simulink model "pickAndPlaceSequence"  (R2019b)
settings: Solver=ode23t  StartTime=0.0  StopTime=40  FixedStep=0.01  MaxStep=0.05  RelTol=1e-3  EnableMultiTasking=on
PreLoadFcn:
  | mdl_puma560
values from neighbouring files (symbols this model uses):
  R = SerialLink(L, 'name', '210F', 'comment', 'six DOF', 'manufacturer', 'FANUC')    [Model_210F.m]
undefined symbols (not defined in the file or in its folder): slcoulomb
libraries: roblocks x14, simulink x7
settings Model: ExtModeTrigMode=oneshot  ExtModeArmWhenConnect=off  Creator=pic  LastModifiedBy=Karl
settings SolverCC: ZeroCrossControl=DisableAll
settings DataIOCC: SaveFormat=Array  SignalLoggingSaveFormat=ModelDataLogs  TimeSaveName=t  OutputSaveName=y  ReturnWorkspaceOutputsName=Rsim
settings OptimizationCC: BlockReduction=off  BooleanDataType=off  ExpressionDepthLimit=2147483647  InitFltsAndDblsToZero=on  LifeSpan=inf
settings DebuggingCC: SaveWithParameterizedLinksMsg=none  UnderspecifiedInitializationDetection=Classic  MergeDetectMultiDrivingBlocksExec=none  SignalResolutionControl=TryResolveAllWithWarning  MultiTaskDSMMsg=warning  MultiTaskCondExecSysMsg=none  FcnCallInpInsideContextMsg=warning  AllowSymbolicDim=off  StateNameClashWarn=warning  SFUnexpectedBacktrackingDiag=warning  SFNoUnconditionalDefaultTransitionDiag=warning  SFExecutionAtInitializationDiag=none  ArithmeticOperatorsInVariantConditions=warning
settings HardwareCC: ProdBitPerPointer=32  ProdBitPerSizeT=32  ProdBitPerPtrDiffT=32  ProdLargestAtomicFloat=None  ProdIntDivRoundTo=Undefined  ProdEndianess=Unspecified  ProdWordSize=32  ProdHWDeviceType=32-bit Generic  TargetUnknown=on
settings ModelReferenceCC: PropagateSignalLabelsOutOfModel=off
settings SFSimCC: SimUseLocalCustomCode=off  CustomCodeUndefinedFunction=UseInterfaceOnly
settings RTWCC: RTWUseLocalCustomCode=off
settings CodeAppCC: StateflowObjectComments=on
settings GRTTargetCC: TargetLangStandard=C89/C90 (ANSI)  ModelReferenceCompliant=off  CompOptLevelCompliant=off  GeneratePreprocessorConditionals=Disable all  CombineOutputUpdateFcns=off  MatFileLogging=off  GRTInterface=on
settings ConfigComp: CovMetricSettings=dw  CovHtmlReporting=on  CovSaveCumulativeToWorkspaceVar=on  CovSaveSingleToWorkspaceVar=on  CovExternalEMLEnable=off

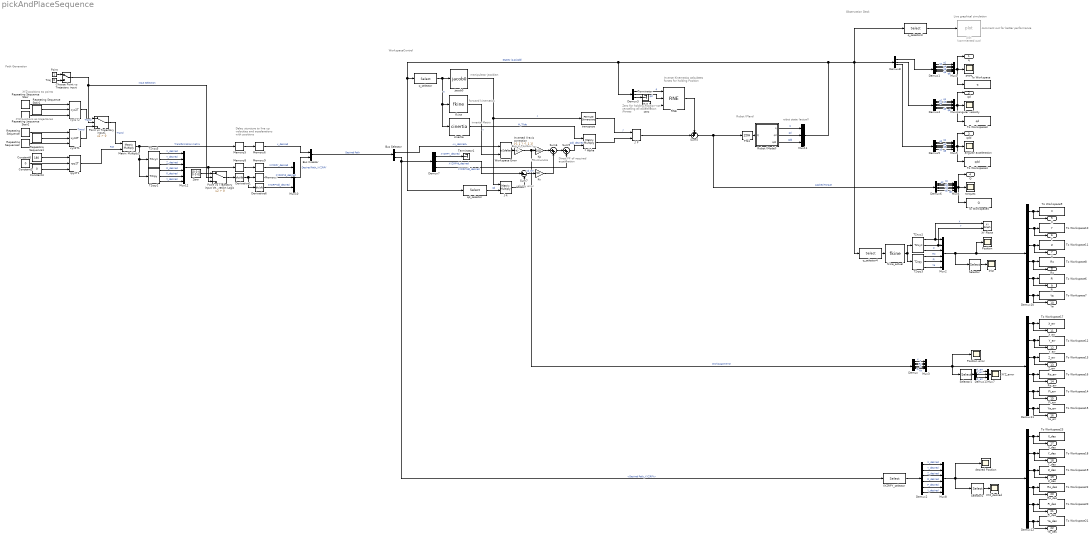
== system pickAndPlaceSequence ==
  note: Live graphical simulation
  note: comment out for better performance
  note: manipulator jacobian
  note: innertia Matrix
  note: forward kinematics
  note: XYZ positions as trajectories
  note: XYZ-positions as points
  note: Delay sturcture to line up velocities and accelerations with positions
  note: position error
  note: velocity error
  note: Direct FF
      | of required
      |  acceleration
  note: PD-strucutre
  note: Inverse Kinematics
      | calculates forces
      | for holding Position
  note: Bug in Toolbox!
  note: WorkspaceControl
  note: Zero for
      | holding Position
      | not cancelling
      | all acceleration
      | /forces
  note: Robot (Plant)
  note: robot state
      | (actual)
  note: Path Generation
  note: Observation Deck
  "* Alpha " : Product  Multiplication=Matrix(*)
  Bus Creator : BusCreator  Inputs=2
  Bus Selector : BusSelector  OutputSignals=x_desired,Desired Path_XYZRPY
  Choose Point vs Trajectory input : ManualSwitch
  Constant1 : Constant  Value=0
  Constant4 : Constant  Value=0
  Constant6 : Constant  Value=180
  Demux{,1..2,4..6,10..12} (9 alike) : Demux  Outputs=6
  Demux{3,7..8,13} (4 alike) : Demux  Outputs=3
  Derivative1 : Derivative
  Derivative6 : Derivative
  "Inverted X-axis correction " : Gain  Gain=[-1 1 1 -1 1 1]
  J q : Product  Multiplication=Matrix(*)
  J' F : Product  Multiplication=Matrix(*)
  Kp : Gain  Gain=100
  Kv : Gain  Gain=50
  Matrix Multiply1 : Product  Multiplication=Matrix(*)
  Memory5 : Memory  InitialCondition=eye(4)  InheritSampleTime=on
  Memory6 : Memory  InitialCondition=eye(4)  InheritSampleTime=on
  Memory7 : Memory  InitialCondition=[0 0 0 0 0 0]  InheritSampleTime=on
  Memory8 : Memory  InitialCondition=[0 0 0 0 0 0]  InheritSampleTime=on
  Memory9 : Memory  InitialCondition=[0 0 0 0 0 0]  InheritSampleTime=on
  Mux{1..6,8,12} (8 alike) : Mux  Inputs=6
  Mux10 : Mux  Inputs=3
  Mux11 : Mux  Inputs=3
  Mux7 : Mux  Inputs=3
  Point : Constant
  Point vs Trajectory input Velocity/Acceleration Logic : Switch  Criteria=u2 > Threshold
  Point vs Trajectory input1 : Switch  Criteria=u2 > Threshold
  Position : Scope
  Position error : Scope
  RNE : roblocks/Arm/RNE  robot=R.nofriction  grav=[0 0 9.81]
  Repeating Sequence : simulink/Sources/Repeating Sequence  rep_seq_t=[0 2 4 6 8 10 12 14 16 18 20 22 24 26 28 30 32]  rep_seq_y=[0.9 0.9 0.9 0.9 1.850 2.250 2.250 2 1.650 2.250 2.250 1.250 0.815 0.815 0.815 0.885 0.9 ]
  Repeating Sequence Stair : simulink/Sources/Repeating Sequence Stair  OutValues=[0.9 0.9 0.9 0.9 1.850 2.250 2.250 2 1.650 2.250 2.250 1.250 0.815 0.815 0.815 0.885 0.9 ]  tsamp=2  OutMin=[]  OutMax=[]  OutDataTypeStr=double  OutputDataTypeScalingMode=double  OutDataType=fixdt(0,8)  ConRadixGroup=Best Precision: Vector-wise  OutScaling=2^-12
  Repeating Sequence Stair1 : simulink/Sources/Repeating Sequence Stair  OutValues=[1.6 1.6 1.6 1 0 0 0 0 0 0 0 0 -1.695 -1.695 -1.695 0.5 1.6]  tsamp=2  OutMin=[]  OutMax=[]  OutDataTypeStr=double  OutputDataTypeScalingMode=double  OutDataType=fixdt(0,8)  ConRadixGroup=Best Precision: Vector-wise  OutScaling=2^-12
  Repeating Sequence Stair2 : simulink/Sources/Repeating Sequence Stair  OutValues=[0.026 -0.05 0.026 0.026 0.14 0.123 0.084 0.13 0.13 0.13 0.155 0.180 -0.17 -0.26 -0.17 0.026 0.026]  tsamp=2  OutMin=[]  OutMax=[]  OutDataTypeStr=double  OutputDataTypeScalingMode=double  OutDataType=fixdt(0,8)  ConRadixGroup=Best Precision: Vector-wise  OutScaling=2^-12
  Repeating Sequence1 : simulink/Sources/Repeating Sequence  rep_seq_t=[0 2 4 6 8 10 12 14 16 18 20 22 24 26 28 30 32]  rep_seq_y=[1.6 1.6 1.6 1 0 0 0 0 0 0 0 0 -1.695 -1.695 -1.695 0.5 1.6]
  Repeating Sequence2 : simulink/Sources/Repeating Sequence  rep_seq_t=[0 2 4 6 8 10 12 14 16 18 20 22 24 26 28 30 32]  rep_seq_y=[0.026 -0.05 0.026 0.026 0.14 0.123 0.084 0.13 0.13 0.13 0.155 0.180 -0.17 -0.26 -0.17 0.026 0.026]
  Robot (Model) : Subsystem  AncestorBlock=roblocks/Arm/Robot  mask{robot=R.nofriction, q0=[0 -pi/4 0 0 -pi/4 0]}
      mask prompts: robot "Robot object"; q0 "Initial state"
      mask help: Rigid-body dynamic model of robot.
      mask init:
      | if isa(robot, 'SerialLink')
      |     rname = robot.name;
      |     %fprintf('**robot name is %s\n', rname);
      | else
      |     rname = '';
      |     n = 0
      | end
      mask Help:
      | Simulates the forward (direct) rigid-body dynamics of the robot described
      | by the given robot object.  For given applied joint torque/force it computes
      | the instaneous joint coordinates, velocities and acclerations.
      | 
      | 
      | <b>Parameters::</b>
      | 
      | robot (SerialLink) a dynamic model of an N-link serial link manipulator
      | q0 (1xN)  Initial joint coordinates
      | 
      | <b>Inputs::</b>
      | 
      | Q (1xN) the generalized joint force (torque or force) required to achieve
      | the motion state (q, qd, qdd).
      | 
      | <b>Outputs::</b>
      | 
      | q (1xN) joint coordinates
      | qd (1xN) joint coordinate velocity
      | qdd (1xN) joint coordinate acceleration
      | 
      | 
      | <b>Notes::</b>
      | 
      | - Required to simulate robot rigid body motion.
      | - Implemented using the recursive Newton-Euler scheme (RNE).
      | - A wrapper for the Toolbox method accel() which in turn depends on the
      |   method rne().
      mask Display:
      | port_label('input', 1, 'Q')
      | port_label('output', 1, 'q')
      | port_label('output', 2, 'qd')
      | port_label('output', 3, 'qdd')
      | text(0.1, 0.9,  rname, 'horizontalAlignment', 'left')
  Selector : Selector  InputPortWidth=6  IndexOptions=Index vector (dialog)  Indices=[1 2 3]  OutputSizes=1
  Selector1 : Selector  InputPortWidth=6  IndexOptions=Index vector (dialog)  Indices=[1 2 3]  OutputSizes=1
  Selector2 : Selector  InputPortWidth=6  IndexOptions=Index vector (dialog)  Indices=[1 2 3]  OutputSizes=1
  Sum5 : Sum  Inputs=++|
  Sum6 : Sum  Inputs=|++
  Sum7 : Sum  Inputs=|+-
  Sum9 : Sum  Inputs=|++
  T2rpy2 : roblocks/Toolbox/T2rpy  sequence=ZYX  degrees=off
  T2rpy3 : roblocks/Toolbox/T2rpy  sequence=ZYX  degrees=off
  T2xyz1 : roblocks/Toolbox/T2xyz
  T2xyz3 : roblocks/Toolbox/T2xyz
  Terminator : Terminator
  Terminator1 : Terminator
  Tfb1 : ZeroOrderHold  SampleTime=0.005
  To Workspace : ToWorkspace  VariableName=q  SaveFormat=Timeseries  SampleTime=-1
  To Workspace10 : ToWorkspace  VariableName=Y  SaveFormat=Timeseries  SampleTime=-1
  To Workspace11 : ToWorkspace  VariableName=Z  SaveFormat=Timeseries  SampleTime=-1
  To Workspace12 : ToWorkspace  VariableName=Y_err  SaveFormat=Timeseries  SampleTime=-1
  To Workspace13 : ToWorkspace  VariableName=Z_err  SaveFormat=Timeseries  SampleTime=-1
  To Workspace14 : ToWorkspace  VariableName=Pi_err  SaveFormat=Timeseries  SampleTime=-1
  To Workspace15 : ToWorkspace  VariableName=Ya_err  SaveFormat=Timeseries  SampleTime=-1
  To Workspace16 : ToWorkspace  VariableName=Ro_err  SaveFormat=Timeseries  SampleTime=-1
  To Workspace17 : ToWorkspace  VariableName=X_err  SaveFormat=Timeseries  SampleTime=-1
  To Workspace18 : ToWorkspace  VariableName=Y_des  SaveFormat=Timeseries  SampleTime=-1
  To Workspace19 : ToWorkspace  VariableName=Z_des  SaveFormat=Timeseries  SampleTime=-1
  To Workspace20 : ToWorkspace  VariableName=Pi_des  SaveFormat=Timeseries  SampleTime=-1
  To Workspace21 : ToWorkspace  VariableName=Ya_des  SaveFormat=Timeseries  SampleTime=-1
  To Workspace22 : ToWorkspace  VariableName=Ro_des  SaveFormat=Timeseries  SampleTime=-1
  To Workspace23 : ToWorkspace  VariableName=X_des  SaveFormat=Timeseries  SampleTime=-1
  To Workspace3 : ToWorkspace  VariableName=qd  SaveFormat=Timeseries  SampleTime=-1
  To Workspace4 : ToWorkspace  VariableName=qdd  SaveFormat=Timeseries  SampleTime=-1
  To Workspace5 : ToWorkspace  VariableName=Q  SaveFormat=Timeseries  SampleTime=-1
  To Workspace6 : ToWorkspace  VariableName=Pi  SaveFormat=Timeseries  SampleTime=-1
  To Workspace7 : ToWorkspace  VariableName=Ya  SaveFormat=Timeseries  SampleTime=-1
  To Workspace8 : ToWorkspace  VariableName=Ro  SaveFormat=Timeseries  SampleTime=-1
  To Workspace9 : ToWorkspace  VariableName=X  SaveFormat=Timeseries  SampleTime=-1
  Traj : Constant  Value=0
  Workspace Error : roblocks/Toolbox/tr2delta
  XY Plane : simulink/Sinks/XY Graph  xmin=-3  xmax=3  ymin=-3  ymax=3  st=-1
  XYZ : Scope
  XYZRPY_selector : Selector  InputPortWidth=18  IndexOptions=Index vector (dialog)  Indices=[1 2 3 4 5 6]  OutputSizes=1
  XYZ_desired : Scope
  XYZ_error : Scope
  "Zero " : Constant  Value=[0 0 0 0 0 0]
  angular acceleration : Scope
  angular velocity : Scope
  "cinertia " : roblocks/Arm/cinertia  robot=R.nofriction
  desired Position : Scope
  "fkine " : roblocks/Arm/fkine  robot=R.nofriction
  fkine_actual : roblocks/Arm/fkine  robot=R.nofriction
  "jacob0 " : roblocks/Arm/jacob0   robot=R.nofriction
  plot : roblocks/Arm/plot  Commented=on  robot=R.nofriction  fps=10  holdplot=on
  pose : Scope
  q_selector : Selector  InputPortWidth=18  IndexOptions=Index vector (dialog)  Indices=[1 2 3 4 5 6]  OutputSizes=1
  q_selector3 : Selector  InputPortWidth=18  IndexOptions=Index vector (dialog)  Indices=[1 2 3 4 5 6]  OutputSizes=1
  q_selector4 : Selector  InputPortWidth=18  IndexOptions=Index vector (dialog)  Indices=[1 2 3 4 5 6]  OutputSizes=1
  qd_selector : Selector  InputPortWidth=18  IndexOptions=Index vector (dialog)  Indices=[7 8 9 10 11 12]  OutputSizes=1
  rpy2T1 : roblocks/Toolbox/rpy2T  sequence=ZYX  degrees=on
  torques : Scope
  transpose : PermuteDimensions
  xyz2T1 : roblocks/Toolbox/xyz2T
  xyz2T2 : roblocks/Toolbox/xyz2T
  zero : Constant  Value=[0 0 0 0 0 0]
  q : Outport  VectorParamsAs1DForOutWhenUnconnected=off
  qd : Outport  Port=2  VectorParamsAs1DForOutWhenUnconnected=off
  qdd : Outport  Port=3  VectorParamsAs1DForOutWhenUnconnected=off
  Q : Outport  Port=4  VectorParamsAs1DForOutWhenUnconnected=off
  X : Outport  Port=5  VectorParamsAs1DForOutWhenUnconnected=off
  Y : Outport  Port=6  VectorParamsAs1DForOutWhenUnconnected=off
  Z : Outport  Port=7
  Ro : Outport  Port=8  VectorParamsAs1DForOutWhenUnconnected=off
  Pi : Outport  Port=9  VectorParamsAs1DForOutWhenUnconnected=off
  Ya : Outport  Port=10
  X_err : Outport  Port=11  VectorParamsAs1DForOutWhenUnconnected=off
  Y_err : Outport  Port=12  VectorParamsAs1DForOutWhenUnconnected=off
  Z_err : Outport  Port=13
  Ro_err : Outport  Port=14  VectorParamsAs1DForOutWhenUnconnected=off
  Pi_err : Outport  Port=15  VectorParamsAs1DForOutWhenUnconnected=off
  Ya_err : Outport  Port=16
  X_des : Outport  Port=17  VectorParamsAs1DForOutWhenUnconnected=off
  Y_des : Outport  Port=18  VectorParamsAs1DForOutWhenUnconnected=off
  Z_des : Outport  Port=19
  Ro_des : Outport  Port=20  VectorParamsAs1DForOutWhenUnconnected=off
  Pi_des : Outport  Port=21  VectorParamsAs1DForOutWhenUnconnected=off
  Ya_des : Outport  Port=22
  wires:
  "jacob0 "/1 -> transpose/1, J q/1  "J"
  "fkine "/1 -> Workspace Error/2  "x"
  zero/1 -> RNE/3
  RNE/1 -> Sum5/1
  J' F/1 -> Sum5/2
  transpose/1 -> J' F/1  "J'"
  "* Alpha "/1 -> J' F/2
  Workspace Error/1 -> "Inverted X-axis correction "/1
  Kv/1 -> Sum6/2
  Sum7/1 -> Kv/1  "xd_err"
  Kp/1 -> Sum6/1
  J q/1 -> Sum7/2
  "cinertia "/1 -> "* Alpha "/1  "M_Tilde"
  Sum6/1 -> Sum9/1
  Demux7/2 -> Sum7/1  "XYZRPYd_desired"
  Sum9/1 -> "* Alpha "/2  "qdd_desired"
  Demux7/3 -> Sum9/2  "XYZRPYdd_desired"
  Memory6/1 -> Bus Creator/1  "x_desired"
  Robot (Model)/3(qdd) -> Mux11/3  "qdd"
  Robot (Model)/2(qd) -> Mux11/2  "qd"
  Robot (Model)/1(q) -> Mux11/1  "q"
  Tfb1/1 -> Robot (Model)/1(Q)
  Demux3/1 -> RNE/1  "q"
  Demux3/2 -> RNE/2  "qd"
  Demux3/3 -> Terminator/1
  qd_selector/1 -> J q/2  "qd"
  Memory8/1 -> Memory9/1
  Derivative1/1 -> Memory7/1, Derivative6/1
  Mux12/1 -> Point vs Trajectory input Velocity/Acceleration Logic/3, Memory8/1
  T2xyz3/2 -> Mux12/2  "Y_desired"
  T2xyz3/3 -> Mux12/3  "Z_desired"
  T2rpy2/2 -> Mux12/5  "P_desired"
  rpy2T1/1 -> Matrix Multiply1/2  "Rot"
  Matrix Multiply1/1 -> T2rpy2/1, T2xyz3/1, Memory5/1  "Transformation matrix"
  Derivative6/1 -> Mux10/3  "XYZRPYdd_desired"
  Memory7/1 -> Mux10/2  "XYZRPYd_desired"
  Point vs Trajectory input1/1 -> Matrix Multiply1/1  "Transl"
  T2rpy2/3 -> Mux12/6  "Y_desired"
  Memory5/1 -> Memory6/1
  Memory9/1 -> Mux10/1  "XYZRPY_desired"
  T2rpy2/1 -> Mux12/4  "R_desired"
  T2xyz3/1 -> Mux12/1  "X_desired"
  q_selector/1 -> "cinertia "/1, "fkine "/1, "jacob0 "/1  "q"
  Demux7/1 -> Terminator1/1  "XYZRPY_desired"
  Bus Selector/2 -> XYZRPY_selector/1, Demux7/1  "<Desired Path_XYZRPY>"
  Demux8/1 -> Demux1/1
  Mux7/1 -> XYZ_error/1
  Demux10/4 -> Ro/1, To Workspace8/1
  Demux10/2 -> Y/1, To Workspace10/1
  Mux11/1 -> Demux8/1, q_selector3/1, q_selector4/1, Demux3/1, qd_selector/1, q_selector/1  "States (q,qd,qdd)"
  q_selector4/1 -> fkine_actual/1
  fkine_actual/1 -> T2rpy3/1, T2xyz1/1
  Demux6/4 -> Mux6/4  "q4"
  Demux2/1 -> Mux8/1  "X_desired"
  Demux2/2 -> Mux8/2  "Y_desired"
  Demux4/3 -> Mux4/3  "q3"
  Demux2/6 -> Mux8/6  "Y_desired"
  Demux6/3 -> Mux6/3  "q3"
  Demux4/1 -> Mux4/1  "q1"
  Sum5/1 -> Tfb1/1, Demux6/1  "Applied Torque"
  Demux4/2 -> Mux4/2  "q2"
  Mux5/1 -> qdd/1, To Workspace4/1, angular acceleration/1
  Demux6/1 -> Mux6/1  "q1"
  Demux4/5 -> Mux4/5  "q5"
  Demux10/3 -> Z/1, To Workspace11/1
  Mux6/1 -> Q/1, To Workspace5/1, torques/1
  Demux6/5 -> Mux6/5  "q5"
  Demux6/6 -> Mux6/6  "q6"
  Demux5/1 -> Mux5/1  "q1"
  Demux10/6 -> Ya/1, To Workspace7/1
  Demux4/4 -> Mux4/4  "q4"
  Demux8/2 -> Demux4/1
  Demux5/6 -> Mux5/6  "q6"
  Demux5/4 -> Mux5/4  "q4"
  Demux1/5 -> Mux1/5  "q5"
  Demux4/6 -> Mux4/6  "q6"
  Demux1/1 -> Mux1/1  "q1"
  Mux1/1 -> q/1, To Workspace/1, pose/1
  Demux1/4 -> Mux1/4  "q4"
  Demux2/4 -> Mux8/4  "R_desired"
  Demux1/2 -> Mux1/2  "q2"
  Demux6/2 -> Mux6/2  "q2"
  Demux2/3 -> Mux8/3  "Z_desired"
  Demux5/3 -> Mux5/3  "q3"
  Demux5/2 -> Mux5/2  "q2"
  Demux2/5 -> Mux8/5  "P_desired"
  Demux1/3 -> Mux1/3  "q3"
  Demux1/6 -> Mux1/6  "q6"
  Selector1/1 -> Demux13/1
  Demux12/1 -> To Workspace23/1, X_des/1
  Demux12/5 -> Pi_des/1, To Workspace20/1
  Demux13/3 -> Mux7/3  "Z_err"
  Demux12/4 -> Ro_des/1, To Workspace22/1
  Demux11/5 -> Pi_err/1, To Workspace14/1
  Demux12/2 -> Y_des/1, To Workspace18/1
  Demux12/3 -> Z_des/1, To Workspace19/1
  Mux4/1 -> qd/1, To Workspace3/1, angular velocity/1
  Demux11/1 -> To Workspace17/1, X_err/1
  Demux11/4 -> Ro_err/1, To Workspace16/1
  Demux11/6 -> Ya_err/1, To Workspace15/1
  T2rpy3/1 -> Mux2/4  "Ro"
  T2rpy3/2 -> Mux2/5  "Pi"
  Demux11/3 -> Z_err/1, To Workspace13/1
  T2xyz1/3 -> Mux2/3  "Z"
  T2xyz1/2 -> XY Plane/2, Mux2/2  "Y"
  q_selector3/1 -> plot/1
  XYZRPY_selector/1 -> Demux2/1
  Selector2/1 -> XYZ_desired/1
  Demux12/6 -> Ya_des/1, To Workspace21/1
  Mux2/1 -> Position/1, Demux10/1, Selector/1
  Demux11/2 -> Y_err/1, To Workspace12/1
  Selector/1 -> XYZ/1
  Demux13/1 -> Mux7/1  "X_err"
  Demux8/3 -> Demux5/1
  Demux5/5 -> Mux5/5  "q5"
  T2rpy3/3 -> Mux2/6  "Ya"
  Demux13/2 -> Mux7/2  "Y_err"
  T2xyz1/1 -> XY Plane/1, Mux2/1  "X"
  Mux8/1 -> Demux12/1, Selector2/1, desired Position/1
  Demux10/5 -> Pi/1, To Workspace6/1
  Demux10/1 -> To Workspace9/1, X/1
  "Inverted X-axis correction "/1 -> Demux/1, Kp/1  "Workspace error"
  Demux/6 -> Mux3/6  "Ya"
  Demux/2 -> Mux3/2  "Y"
  Demux/4 -> Mux3/4  "Ro"
  Demux/5 -> Mux3/5  "Pi"
  Demux/1 -> Mux3/1  "X"
  Demux/3 -> Mux3/3  "Z"
  Mux3/1 -> Selector1/1, Position error/1, Demux11/1
  Bus Creator/1 -> Bus Selector/1  "Desired Path"
  Mux10/1 -> Bus Creator/2  "Desired Path_XYZRPY"
  Bus Selector/1 -> Workspace Error/1  "<x_desired>"
  Constant6/1 -> rpy2T1/1
  Constant1/1 -> rpy2T1/2
  Constant4/1 -> rpy2T1/3
  Repeating Sequence Stair2/1 -> xyz2T2/3
  Repeating Sequence Stair1/1 -> xyz2T2/2
  Repeating Sequence Stair/1 -> xyz2T2/1
  Repeating Sequence/1 -> xyz2T1/1
  Repeating Sequence2/1 -> xyz2T1/3
  Repeating Sequence1/1 -> xyz2T1/2
  xyz2T2/1 -> Point vs Trajectory input1/1  "Transl"
  xyz2T1/1 -> Point vs Trajectory input1/3  "Transl"
  Point vs Trajectory input Velocity/Acceleration Logic/1 -> Derivative1/1
  Point/1 -> Choose Point vs Trajectory input/1
  Traj/1 -> Choose Point vs Trajectory input/2
  Choose Point vs Trajectory input/1 -> Point vs Trajectory input Velocity/Acceleration Logic/2, Point vs Trajectory input1/2  "Input Selection"
  "Zero "/1 -> Point vs Trajectory input Velocity/Acceleration Logic/1

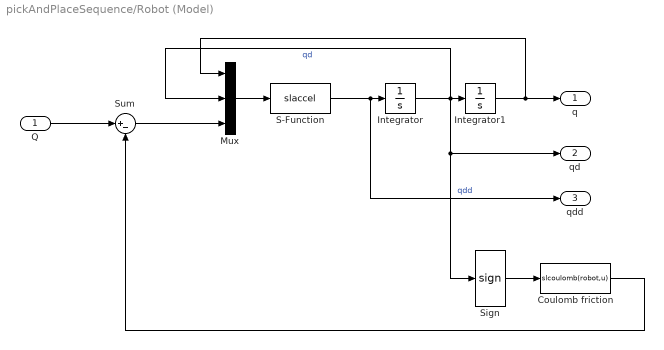
== system pickAndPlaceSequence/Robot (Model) ==
  Q : Inport
  Coulomb friction : MATLABFcn  MATLABFcn=slcoulomb(robot,u)  OutputDimensions=[robot.n 1]  Output1D=off
  Integrator : Integrator
  Integrator1 : Integrator  InitialCondition=q0
  Mux : Mux  Inputs=3
  S-Function : S-Function  FunctionName=slaccel  Parameters=robot  SFunctionDeploymentMode=off  EnableBusSupport=off
  Sign : Signum
  Sum : Sum  Inputs=|+-
  q : Outport  VectorParamsAs1DForOutWhenUnconnected=off
  qd : Outport  Port=2  VectorParamsAs1DForOutWhenUnconnected=off
  qdd : Outport  Port=3  VectorParamsAs1DForOutWhenUnconnected=off
  wires:
  S-Function/1 -> qdd/1, Integrator/1  "qdd"
  Mux/1 -> S-Function/1
  Integrator/1 -> Sign/1, qd/1, Integrator1/1, Mux/2  "qd"
  Integrator1/1 -> q/1, Mux/1
  Q/1 -> Sum/1
  Sum/1 -> Mux/3
  Coulomb friction/1 -> Sum/2
  Sign/1 -> Coulomb friction/1
